simulink model "model"  (R2021a)
settings: Solver=VariableStepAuto  StartTime=0.0  StopTime=10.0  RelTol=1e-3
libraries: simulink x6, sharedutil x5, aerolibutil x1
(part 2 of 2)

== matlab function model/dynamik/Triggered Subsystem/MATLAB Function1 ==
  settings: updateMethod=DISCRETE
  data: u input; v input; w input; p input; q input; r input; x input; y input; z input; phi input; theta input; psi input; xdot output; n input; mp input; rp input; V_c input; beta_c input; F_1 input; F_2 input; alpha_1 input; alpha_2 input; U_tot output
function [xdot,U_tot] = otter(u, v, w, p, q, r, x, y, z, phi, theta, psi,n,mp,rp,V_c,beta_c,F_1,F_2,alpha_1,alpha_2)
% [xdot,U] = otter(x,n,mp,rp,V_c,beta_c) returns the speed U in m/s (optionally) 
% and the time derivative of the state vector: 
x = [u v w p q r x y z phi theta psi]'; 
% for the Maritime Robotics Otter USV, see www.maritimerobotics.com. 
% The length of the USV is L = 2.0 m, while the state vector is defined as:
%
%  u:     surge velocity          (m/s)
%  v:     sway velocity           (m/s)
%  w:     heave velocity          (m/s)
%  p:     roll velocity           (rad/s)
%  q:     pitch velocity          (rad/s)
%  r:     yaw velocity            (rad/s)
%  x:     position in x direction (m)
%  y:     position in y direction (m)
%  z:     position in z direction (m)
%  phi:   roll angle              (rad)
%  theta: pitch angle             (rad)
%  psi:   yaw angle               (rad)
%
% The other inputs are:
%
% n = [ n(1) n(2) ]' where
%    n(1): propeller shaft speed, left (rad/s)
%    n(2): propeller shaft speed, right (rad/s)
%
% mp = payload mass (kg), maximum 45 kg
%  rp = [xp, yp, zp]' (m) is the location of the payload w.r.t. the CO
%  V_c:     current speed (m/s)
%  beta_c:  current direction (rad)
%
% See, ExOtter.m and demoOtterUSVHeadingControl.slx
%
% Author:    Thor I. Fossen
% Date:      2019-07-17
% Revisions: 2021-04-25 added call to new function crossFlowDrag.m
%            2021-06-21 Munk moment in yaw is neglected
%            2021-07-22 Added a new state for the trim moment
%            2021-12-17 New method Xudot = -addedMassSurge(m,L,rho) 

% Check of input and state dimensions
if (length(x) ~= 12),error('x vector must have dimension 12!'); end
if (length(n) ~= 2),error('n vector must have dimension 2!'); end

% trim: theta = -7.5 deg corresponds to 13.5 cm less height aft maximum load
trim_setpoint = 280;

% trim_setpoint is a step input, which is filtered using the state trim_moment
persistent trim_moment;

if isempty(trim_moment)
   trim_moment = 0;
end

% % Main data
% g   = 9.81;         % acceleration of gravity (m/s^2)
% rho = 1025;         % density of water
% L = 2.0;            % length (m)
% B = 1.08;           % beam (m)
% m = 55.0;           % mass (kg)
% rg = [0.2 0 -0.2]'; % CG for hull only (m)
% R44 = 0.4 * B;      % radii of gyrations (m)
% R55 = 0.25 * L;
% R66 = 0.25 * L;
% T_yaw = 1;          % time constant in yaw (s)
% Umax = 6 * 0.5144;  % max forward speed (m/s)
% 
% % Data for one pontoon
% B_pont  = 0.25;     % beam of one pontoon (m)
% y_pont  = 0.395;    % distance from centerline to waterline area center (m)
% Cw_pont = 0.75;     % waterline area coefficient (-)
% Cb_pont = 0.4;      % block coefficient, computed from m = 55 kg


% Main data
g   = 9.81;         % acceleration of gravity (m/s^2)
rho = 1025;         % density of water
L = 6.969;          % length (m)
B = 3.465;          % beam (m)
m = 775;            % mass (kg)
rg = [0 0 -0.044]'; % CG for hull only (m)
% R44 = 0.4 * B;    % radii of gyrations (m)
% R55 = 0.25 * L;
% R66 = 0.25 * L;
R44 = 0.78934 * B; %0.62879*B;  % radii of gyrations (m)
R55 = 0.18482 * L; %0.24044*L; 
R66 = 0.23465 * L; %0.38756*L; 
T_yaw = 1 ;%2.5;%1;          % time constant in yaw (s)
Umax = 8 * 0.5144;  % max forward speed (m/s)


% Data for one pontoon
B_pont  = 0.696;    % beam of one pontoon (m)
y_pont  = 1.3395;   % distance from centerline to waterline area center (m)
Cw_pont = 0.75;     % waterline area coefficient (-)
%Cb_pont = 0.4;      % block coefficient, computed from m = 55 kg
Cb_pont = 0.375; % overslagsberegning af Cb


%%%%%%%%%%%%%%%%%%%%%%%%%%%%%%%%%%%%%%%%%%%%%%%%%%%%%%%%%%%%%%%%%%%%%%%%%%

% State and current variables
nu = x(1:6);                                % velocities [u v w p q r]
nu1 = x(1:3);                               % velocities [u v w]
nu2 = x(4:6);                               % velocities [p q r]
eta = x(7:12);                              % positions [x y z phi theta psi ]
U = sqrt(nu(1)^2 + nu(2)^2 + nu(3)^2);      % speed
u_c = V_c * cos(beta_c - eta(6));           % current surge velocity
v_c = V_c * sin(beta_c - eta(6));           % current sway velocity
nu_r = nu - [u_c v_c 0 0 0 0]';             % relative velocity vector

% Inertia dyadic, volume displacement and draft
nabla = (m+mp)/rho;                         % volume
T = nabla / (2 * Cb_pont * B_pont*L);       % draft
Ig_CG = m * diag([R44^2, R55^2, R66^2]);    % only hull in CG
rg = (m*rg + mp*rp)/(m+mp);           % CG location corrected for payload
Ig = Ig_CG - m * Smtrx(rg)^2 - mp * Smtrx(rp)^2;  % hull + payload in CO

% Experimental propeller data including lever arms
l1 = -y_pont;                           % lever arm, left propeller (m)
l2 = y_pont;                            % lever arm, right propeller (m)
k_pos = 0.02216/2;                      % Positive Bollard, one propeller 
k_neg = 0.01289/2;                      % Negative Bollard, one propeller 
n_max = 300.42; %sqrt((0.5*24.4 * g)/k_pos);    % maximum propeller rev. (rad/s)
n_min = -300.42; %-sqrt((0.5*13.6 * g)/k_neg);    % minimum propeller rev. (rad/s)
F_max = 1000;
F_min = -1000;

% MRB and CRB (Fossen 2021)
I3 = eye(3);
O3 = zeros(3,3);

MRB_CG = [ (m+mp) * I3  O3
           O3           Ig ];
CRB_CG = [ (m+mp) * Smtrx(nu2)         O3
           O3               -Smtrx(Ig*nu2)  ];

H = Hmtrx(rg);              % Transform MRB and CRB from the CG to the CO 
MRB = H' * MRB_CG * H;
CRB = H' * CRB_CG * H;

% Hydrodynamic added mass (best practise)
Xudot = -addedMassSurge(m,L,rho);   
Yvdot = -1.5 * m;
Zwdot = -1.0 * m;
Kpdot = -0.2 * Ig(1,1);
Mqdot = -0.8 * Ig(2,2);
Nrdot = -1.7 * Ig(3,3);




MA = -diag([Xudot, Yvdot, Zwdot, Kpdot, Mqdot, Nrdot]);   
CA  = m2c(MA, nu_r);
CA(6,1) = 0; % Assume that the Munk moment in yaw can be neglected
CA(6,2) = 0; % These terms, if nonzero, must be balanced by adding nonlinear damping

% System mass and Coriolis-centripetal matrices
M = MRB + MA;
C = CRB + CA;

% Hydrostatic quantities (Fossen 2021)
Aw_pont = Cw_pont * L * B_pont;    % waterline area, one pontoon 
I_T = 2 * (1/12)*L*B_pont^3 * (6*Cw_pont^3/((1+Cw_pont)*(1+2*Cw_pont)))...
    + 2 * Aw_pont * y_pont^2;
I_L = 0.8 * 2 * (1/12) * B_pont * L^3;
KB = (1/3)*(5*T/2 - 0.5*nabla/(L*B_pont) );
BM_T = I_T/nabla;       % BM values
BM_L = I_L/nabla;
KM_T = KB + BM_T;       % KM values
KM_L = KB + BM_L;
KG = T - rg(3);
GM_T = KM_T - KG;       % GM values
GM_L = KM_L - KG;

G33 = rho * g * (2 * Aw_pont);      % spring stiffness
G44 = rho * g *nabla * GM_T;
G55 = rho * g *nabla * GM_L;

G_CF = diag([0 0 G33 G44 G55 0]);   % spring stiffness matrix in the CF
LCF = -0.2;
H = Hmtrx([LCF 0 0]);               % transform G_CF from the CF to the CO 
G = H' * G_CF * H;

% Natural frequencies
w3 = sqrt( G33/M(3,3) );         
w4 = sqrt( G44/M(4,4) );
w5 = sqrt( G55/M(5,5) );

% Linear damping terms (hydrodynamic derivatives)
    
if nu_r(1) < 1 && nu_r(1) > -1
%     if nu_r(1) < 0.5
%         Xu = -130;
%     else
    Xu = -130;
%    end
else 
     Xu = -51.3;
end

%Xu = -1.5 ;% -51.3;% -775; %(-24.4 * g / Umax);           % specified using the maximum speed  
Yv = -51.3;
Zw = -2 * 0.3 *w3 * M(3,3);      % specified using relative damping factors
Kp = -2 * 0.2 *w4 * M(4,4);
Mq = -2 * 0.4 *w5 * M(5,5);
Nr = -M(6,6) / T_yaw;            % specified using the time constant in T_yaw

% % Control forces and moments - with propeller revolution saturation 
% Thrust = zeros(2,1);
% for i = 1:1:2
%     if n(i) > n_max              % saturation, physical limits
%        n(i) = n_max; 
%     elseif n(i) < n_min
%        n(i) = n_min; 
%     end
%     
%    if n(i) > 0                          
%      Thrust(i) = k_pos * n(i)*abs(n(i));    % positive thrust (N) 
%    else
%      Thrust(i) = k_neg * n(i)*abs(n(i));    % negative thrust (N) 
%    end
% end
% 
% % Control forces and moments
% tau = [Thrust(1) + Thrust(2) 0 0 0 0 -l1 * Thrust(1) - l2 * Thrust(2) ]';

% Control forces and moments - with propeller revolution saturation 

if F_1 > F_max              % saturation, physical limits
  F_1 = F_max; 
elseif F_1 < F_min
  F_1 = F_min; 
end
if F_2 > F_max              % saturation, physical limits
  F_2 = F_max; 
elseif F_1 < F_min
  F_2 = F_min; 
end

% Control forces and moments
tau = [F_1*cos(alpha_1)+F_2*cos(alpha_2) F_1*sin(alpha_1)+F_2*sin(alpha_2) 0 0 0 F_1*y_pont*cos(alpha_1)-F_2*y_pont*cos(alpha_2)]';



% Linear damping using relative velocities + nonlinear yaw damping
Xh = Xu * nu_r(1);
Yh = Yv * nu_r(2); 
Zh = Zw * nu_r(3);
Kh = Kp * nu_r(4);
Mh = Mq * nu_r(5);
%Nh = Nr * (1 + 10 * abs(nu_r(6))) * nu_r(6);
Nh = Nr * (1 + 1 * abs(nu_r(6))) * nu_r(6);


tau_damp = [Xh Yh Zh Kh Mh Nh]';

% Strip theory: cross-flow drag integrals for Yh and Nh
tau_crossflow = crossFlowDrag(L,B_pont,T,nu_r);

% Ballast
g_0 = [0 0 0 0 trim_moment 0]';

% Kinematics
J = eulerang(eta(4),eta(5),eta(6));


%lig = tau + tau_damp + tau_crossflow - C * nu_r - G * eta - g_0   % til at
%finde forces

% Time derivative of the state vector - numerical integration; see ExOtter.m  
xdot = [ M \ ( tau + tau_damp + tau_crossflow - C * nu_r - G * eta - g_0)
         J * nu ];  
     
trim_moment = trim_moment + 0.05 * (trim_setpoint - trim_moment);
U_tot = U;
end

== matlab function model/dynamik/Dynamic Model1/Construct Matrices/M/M-matrice ==
  data: m input; M_out output; x_g input; y_g input; I_z input; Xu_dot input; Yv_dot input; Yr_dot input; Nr_dot input; Nv_dot input
function M_out = fcn(m,x_g,y_g,I_z, Xu_dot, Yv_dot, Yr_dot, Nr_dot,Nv_dot)

%      M_RB = [m ,   0   , -m*y_g;
%              0 ,   m   ,  m*x_g;
%              -m*y_g , m*x_g ,    I_z];
%          
%      M_A = [-Xu_dot ,      0   ,    0   ;
%                0    ,  -Yv_dot , -Yr_dot;
%                0    ,  -Nv_dot , -Nr_dot];
%          
         

    M_RB = [m ,   0   ,    0;
            0 ,   m   ,  m*x_g;
            0 , m*x_g ,   I_z];


    M_A = [-Xu_dot ,      0   ,    0   ;
              0    ,  -Yv_dot , -Yr_dot;
              0    ,  -Yr_dot , -Nr_dot];
   



    M = M_A + M_RB;

    m_inv = inv(M);


M_out = M;
